simulink model "REV3"  (R2023b)
settings: Solver=ode8  StartTime=0.0  StopTime=inf  FixedStep=0.0001  RelTol=1e-3
settings Model: DataDictionary=rev3_data.sldd  Creator=rebek  LastModifiedBy=mjmag

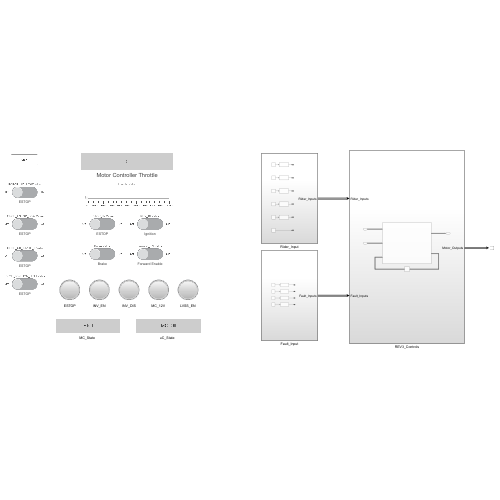
[thumbnail: Simulink's stored preview of the top-level diagram]
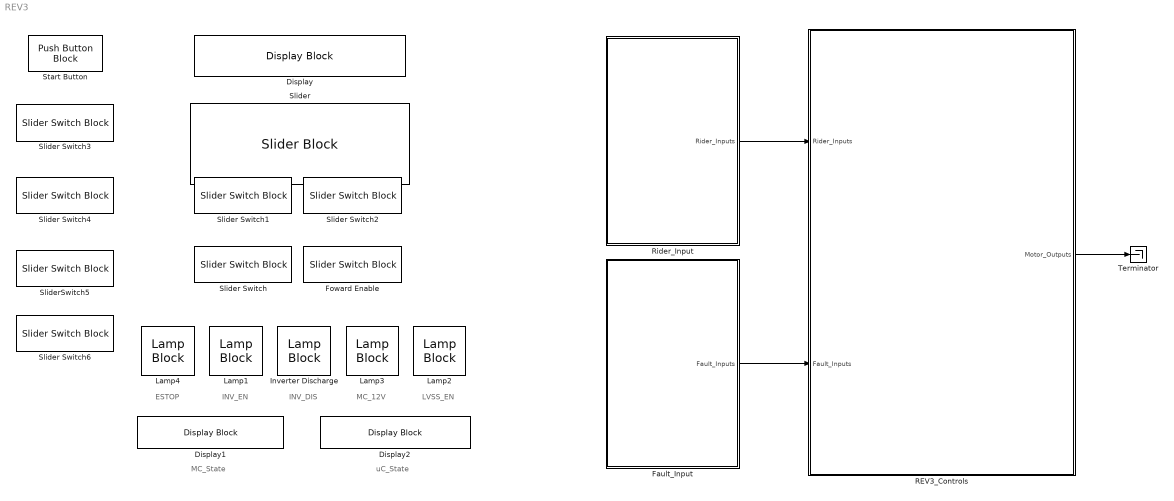
== system REV3 ==
  note: MC_State
  note: LVSS_EN
  note: INV_EN
  note: INV_DIS
  note: MC_12V
  note: uC_State
  note: ESTOP
  Display : DisplayBlock  LabelPosition=Hide  Transparency=1
      settings: AttributesFormatString=Motor Controller Throttle
  Display1 : DisplayBlock  LabelPosition=Hide  Transparency=1
  Display2 : DisplayBlock  LabelPosition=Hide  Transparency=1
  Fault_Input : Subsystem
  Foward Enable : SliderSwitchBlock
      settings: Values={{'Off', 'On'}, [0 1]}
      settings: AttributesFormatString=Forward Enable
  Inverter Discharge : LampBlock  LabelPosition=Hide
  Lamp{1..4} (4 alike) : LampBlock  LabelPosition=Hide
  REV3_Controls : Subsystem
  Rider_Input : Subsystem
  Slider : SliderBlock  ScaleMax=4000
  Slider Switch{,1..4,6} (6 alike) : SliderSwitchBlock
      settings: Values={{'Off', 'On'}, [0 1]}
      Slider Switch settings: AttributesFormatString=Brake
      Slider Switch1 settings: AttributesFormatString=ESTOP
      Slider Switch2 settings: AttributesFormatString=Ignition
      Slider Switch3 settings: AttributesFormatString=ESTOP
      Slider Switch4 settings: AttributesFormatString=ESTOP
      Slider Switch6 settings: AttributesFormatString=ESTOP
  SliderSwitch5 : SliderSwitchBlock
      settings: Values={{'Off', 'On'}, [0 1]}
      settings: AttributesFormatString=ESTOP
  Start Button : PushButtonBlock  ButtonText=Start  OffValue=0.000000
  Terminator : Terminator
  wires:
  Rider_Input/1(Rider_Inputs) -> REV3_Controls/1(Rider_Inputs)
  Fault_Input/1(Fault_Inputs) -> REV3_Controls/2(Fault_Inputs)
  REV3_Controls/1(Motor_Outputs) -> Terminator/1

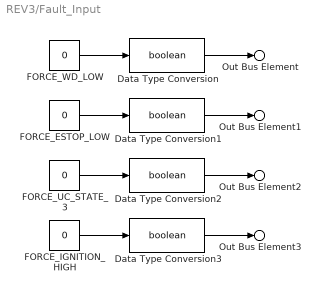
== system REV3/Fault_Input ==
  Data Type Conversion{,1..3} (4 alike) : DataTypeConversion  OutDataTypeStr=boolean  SaturateOnIntegerOverflow=off  RndMeth=Floor
  FORCE_ESTOP_LOW : Constant  Value=0
  FORCE_IGNITION_HIGH : Constant  Value=0
  FORCE_UC_STATE_3 : Constant  Value=0
  FORCE_WD_LOW : Constant  Value=0
  Out Bus Element : Outport  PortName=Fault_Inputs  Element=Force_WD_Low
  Out Bus Element1 : Outport  PortName=Fault_Inputs  Element=Force_Estop_Low
  Out Bus Element2 : Outport  PortName=Fault_Inputs  Element=Force_UC_State_3
  Out Bus Element3 : Outport  PortName=Fault_Inputs  Element=Force_Ignition_High
  wires:
  FORCE_WD_LOW/1 -> Data Type Conversion/1
  FORCE_ESTOP_LOW/1 -> Data Type Conversion1/1
  FORCE_UC_STATE_3/1 -> Data Type Conversion2/1
  FORCE_IGNITION_HIGH/1 -> Data Type Conversion3/1
  Data Type Conversion/1 -> Out Bus Element/1
  Data Type Conversion1/1 -> Out Bus Element1/1
  Data Type Conversion2/1 -> Out Bus Element2/1
  Data Type Conversion3/1 -> Out Bus Element3/1

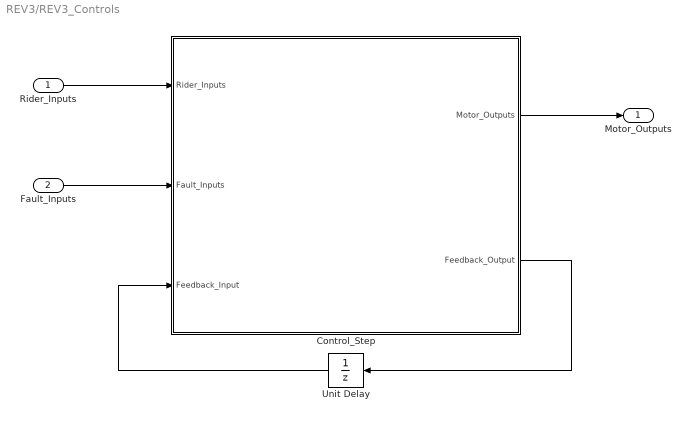
== system REV3/REV3_Controls ==
  Rider_Inputs : Inport
  Fault_Inputs : Inport  Port=2
  Control_Step : Subsystem
  Unit Delay : UnitDelay  SampleTime=-1  HasFrameUpgradeWarning=on
  Motor_Outputs : Outport
  wires:
  Rider_Inputs/1 -> Control_Step/1(Rider_Inputs)
  Fault_Inputs/1 -> Control_Step/2(Fault_Inputs)
  Unit Delay/1 -> Control_Step/3(Feedback_Input)
  Control_Step/1(Motor_Outputs) -> Motor_Outputs/1
  Control_Step/2(Feedback_Output) -> Unit Delay/1

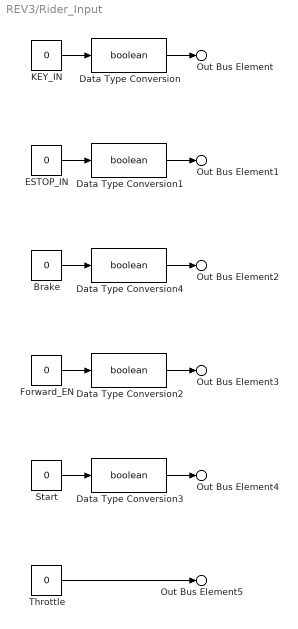
== system REV3/Rider_Input ==
  Brake : Constant  Value=0
  Data Type Conversion{,1..4} (5 alike) : DataTypeConversion  OutDataTypeStr=boolean  SaturateOnIntegerOverflow=off  RndMeth=Floor
  ESTOP_IN : Constant  Value=0
  Forward_EN : Constant  Value=0
  KEY_IN : Constant  Value=0
  Start : Constant  Value=0
  Throttle : Constant  Value=0  OutDataTypeStr=int16
  Out Bus Element : Outport  PortName=Rider_Inputs  Element=Key_In
  Out Bus Element1 : Outport  PortName=Rider_Inputs  Element=Estop_In
  Out Bus Element2 : Outport  PortName=Rider_Inputs  Element=Brake
  Out Bus Element3 : Outport  PortName=Rider_Inputs  Element=Forward_EN
  Out Bus Element4 : Outport  PortName=Rider_Inputs  Element=Start
  Out Bus Element5 : Outport  PortName=Rider_Inputs  Element=Throttle
  wires:
  KEY_IN/1 -> Data Type Conversion/1
  Brake/1 -> Data Type Conversion4/1
  Data Type Conversion4/1 -> Out Bus Element2/1
  Data Type Conversion2/1 -> Out Bus Element3/1
  Data Type Conversion/1 -> Out Bus Element/1
  Forward_EN/1 -> Data Type Conversion2/1
  Data Type Conversion3/1 -> Out Bus Element4/1
  ESTOP_IN/1 -> Data Type Conversion1/1
  Throttle/1 -> Out Bus Element5/1
  Data Type Conversion1/1 -> Out Bus Element1/1
  Start/1 -> Data Type Conversion3/1

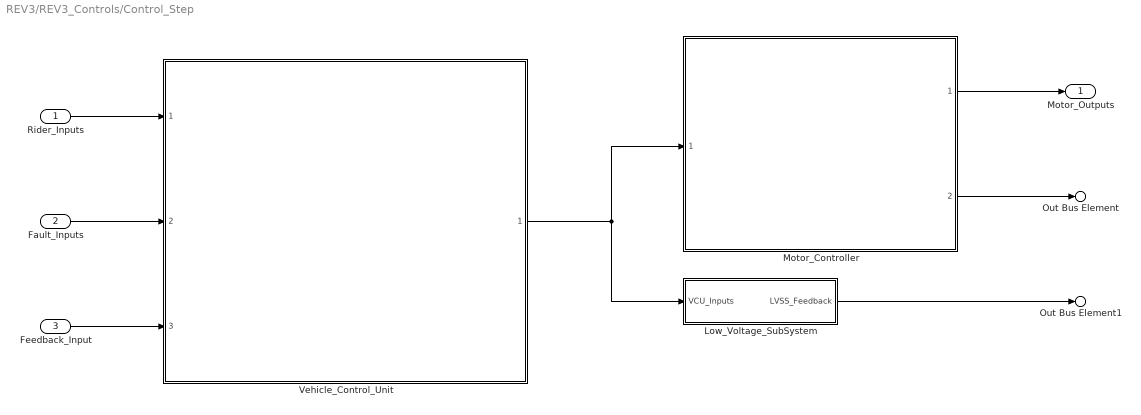
== system REV3/REV3_Controls/Control_Step ==
  Rider_Inputs : Inport
  Fault_Inputs : Inport  Port=2
  Feedback_Input : Inport  Port=3
  Low_Voltage_SubSystem : Subsystem
  Motor_Controller : Subsystem  ReferencedSubsystem=PM100DXR_MC
  Vehicle_Control_Unit : Subsystem  ReferencedSubsystem=VCU
  Motor_Outputs : Outport
  Out Bus Element : Outport  Port=2  PortName=Feedback_Output  Element=MC_Feedback
  Out Bus Element1 : Outport  Port=2  PortName=Feedback_Output  Element=LVSS_Feedback
  wires:
  Vehicle_Control_Unit/1 -> Low_Voltage_SubSystem/1(VCU_Inputs), Motor_Controller/1
  Rider_Inputs/1 -> Vehicle_Control_Unit/1
  Fault_Inputs/1 -> Vehicle_Control_Unit/2
  Motor_Controller/2 -> Out Bus Element/1
  Motor_Controller/1 -> Motor_Outputs/1
  Feedback_Input/1 -> Vehicle_Control_Unit/3
  Low_Voltage_SubSystem/1(LVSS_Feedback) -> Out Bus Element1/1

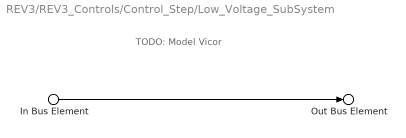
== system REV3/REV3_Controls/Control_Step/Low_Voltage_SubSystem ==
  note: TODO: Model Vicor
  In Bus Element : Inport  PortName=VCU_Inputs  Element=LVSS_Outputs.LVSS_EN
  Out Bus Element : Outport  PortName=LVSS_Feedback  Element=LVSS_ON
  wires:
  In Bus Element/1 -> Out Bus Element/1
